simulink model "simulink_simulacion"  (R2017b)
settings: Solver=VariableStepAuto  StartTime=0.0  StopTime=10.0  RelTol=1e-3
settings Model: Creator=kiriost  LastModifiedBy=kiriost

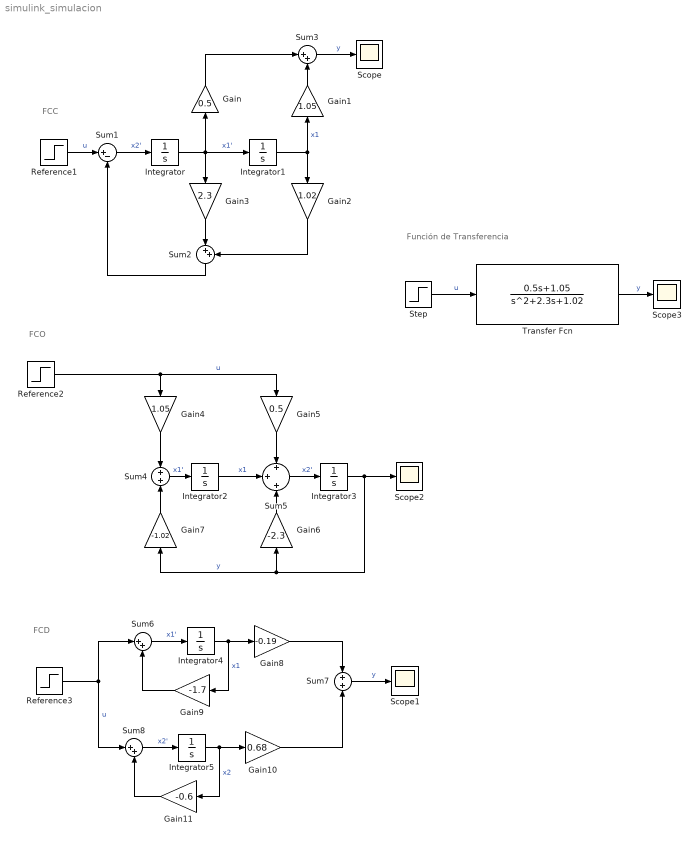
== system simulink_simulacion ==
  note: FCD
  note: FCO
  note: FCC
  note: Función de Transferencia
  Gain : Gain  Gain=0.5
  Gain1 : Gain  Gain=1.05
  Gain10 : Gain  Gain=0.68
  Gain11 : Gain  Gain=-0.6
  Gain2 : Gain  Gain=1.02
  Gain3 : Gain  Gain=2.3
  Gain4 : Gain  Gain=1.05
  Gain5 : Gain  Gain=0.5
  Gain6 : Gain  Gain=-2.3
  Gain7 : Gain  Gain=-1.02
  Gain8 : Gain  Gain=-0.19
  Gain9 : Gain  Gain=-1.7
  Integrator{,1..5} (6 alike) : Integrator
  Reference1 : Step  SampleTime=0
  Reference2 : Step  SampleTime=0
  Reference3 : Step  SampleTime=0
  Scope{,1..3} (4 alike) : Scope
  Step : Step  SampleTime=0
  Sum1 : Sum  Inputs=|+-
  Sum{2..3,6,8} (4 alike) : Sum  Inputs=|++
  Sum4 : Sum  Inputs=+|+
  Sum5 : Sum  Inputs=+|+|+
  Sum7 : Sum
  Transfer Fcn : TransferFcn  Numerator=[0.5 1.05]  Denominator=[1 2.3 1.02]
  wires:
  Sum4/1 -> Integrator2/1  "x1'"
  Sum6/1 -> Integrator4/1  "x1'"
  Integrator2/1 -> Sum5/2  "x1"
  Reference3/1 -> Sum8/1, Sum6/1  "u"
  Integrator4/1 -> Gain9/1, Gain8/1  "x1"
  Gain1/1 -> Sum3/2
  Sum7/1 -> Scope1/1  "y"
  Gain9/1 -> Sum6/2
  Gain7/1 -> Sum4/2
  Gain/1 -> Sum3/1
  Reference2/1 -> Gain5/1, Gain4/1  "u"
  Gain2/1 -> Sum2/2
  Sum8/1 -> Integrator5/1  "x2'"
  Gain11/1 -> Sum8/2
  Integrator5/1 -> Gain11/1, Gain10/1  "x2"
  Gain3/1 -> Sum2/1
  Gain10/1 -> Sum7/2
  Gain4/1 -> Sum4/1
  Sum3/1 -> Scope/1  "y"
  Gain5/1 -> Sum5/1
  Integrator1/1 -> Gain1/1, Gain2/1  "x1"
  Reference1/1 -> Sum1/1  "u"
  Gain6/1 -> Sum5/3
  Sum5/1 -> Integrator3/1  "x2'"
  Step/1 -> Transfer Fcn/1  "u"
  Integrator3/1 -> Gain6/1, Gain7/1, Scope2/1  "y"
  Gain8/1 -> Sum7/1
  Sum2/1 -> Sum1/2
  Transfer Fcn/1 -> Scope3/1  "y"
  Integrator/1 -> Gain3/1, Integrator1/1, Gain/1  "x1'"
  Sum1/1 -> Integrator/1  "x2'"
